simulink model "controllo_ss_PP_Luenberger"  (R2023b)
settings: Solver=VariableStepAuto  StartTime=0.0  StopTime=10  RelTol=1e-3
values from neighbouring files (symbols this model uses):
  C = 3212.6*(s+39.02)/(s+244.3)    [controllore_mag_lin.m]
undefined symbols (not defined in the file or in its folder): A, A_ob, B, B_ob, C_ob, D, D_ob, Ken_eta, Ken_x
settings Model: Creator=Pronto all'uso  LastModifiedBy=Pronto all'uso

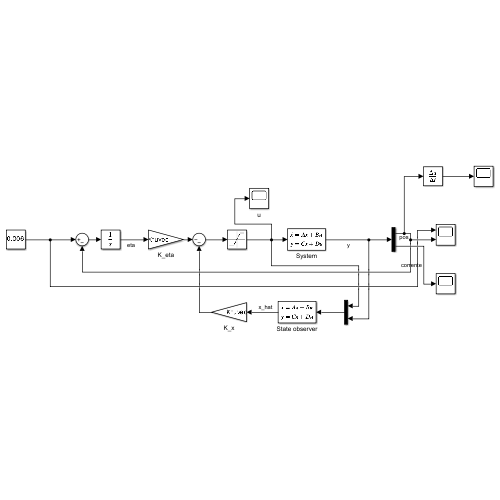
[thumbnail: Simulink's stored preview of the top-level diagram]
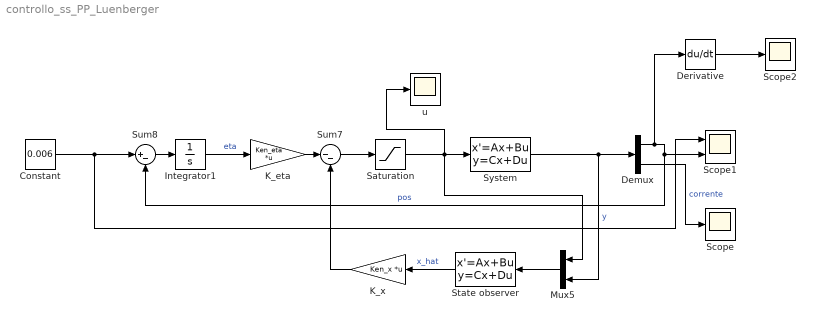
== system controllo_ss_PP_Luenberger ==
  Constant : Constant  Value=0.006
  Demux : Demux  Outputs=2
  Derivative : Derivative
  Integrator1 : Integrator
  K_eta : Gain  Gain=Ken_eta  Multiplication=Matrix(K*u) (u vector)
  K_x : Gain  Gain=Ken_x  Multiplication=Matrix(K*u) (u vector)
  Mux5 : Mux  Inputs=2
  Saturation : Saturate  UpperLimit=23  LowerLimit=-23
  Scope : Scope
  Scope1 : Scope  NumInputPorts=2
  Scope2 : Scope
  State observer : StateSpace  A=A_ob  B=B_ob  C=C_ob  D=D_ob  InitialCondition=[0.005;0;0]  ParameterTunability=Unconstrained
  Sum7 : Sum  Inputs=|--
  Sum8 : Sum  Inputs=|+-
  System : StateSpace  A=A  B=B  C=C  D=D  InitialCondition=[0.005; 0;0]  ParameterTunability=Unconstrained
  u : Scope
  wires:
  Integrator1/1 -> K_eta/1  "eta"
  K_x/1 -> Sum7/2
  Sum8/1 -> Integrator1/1
  K_eta/1 -> Sum7/1
  System/1 -> Demux/1, Mux5/2  "y"
  State observer/1 -> K_x/1  "x_hat"
  Mux5/1 -> State observer/1
  Demux/1 -> Derivative/1, Scope1/2, Sum8/2  "pos"
  Demux/2 -> Scope/1  "corrente"
  Constant/1 -> Scope1/1, Sum8/1
  Sum7/1 -> Saturation/1
  Saturation/1 -> Mux5/1, u/1, System/1
  Derivative/1 -> Scope2/1
